simulink model "smib_53_start"  (Simulink 3.00)
settings: Solver=ode3  StartTime=0.0  StopTime=15  FixedStep=1e-4  MaxStep=1e-4  RelTol=1e-4
values from neighbouring files (symbols this model uses):
  D = 0.01    [MODEL_WORKSPACE.mat]    (also in MODEL_WORKSPACE_53.mat; WS.mat)
  J = 20    [MODEL_WORKSPACE.mat]    (also in MODEL_WORKSPACE_53.mat; WS.mat)
  Rf = 0.00246    [MODEL_WORKSPACE.mat]    (also in MODEL_WORKSPACE_53.mat = 0.0025; WS.mat = 0.0025)
  Tdo = 3    [MODEL_WORKSPACE.mat]    (also in MODEL_WORKSPACE_53.mat; WS.mat)
  X = 0.4    [MODEL_WORKSPACE.mat]    (also in MODEL_WORKSPACE_53.mat; WS.mat)
  Xd = 1    [MODEL_WORKSPACE.mat]    (also in MODEL_WORKSPACE_53.mat; WS.mat)
  Xdp = 0.25    [MODEL_WORKSPACE.mat]    (also in MODEL_WORKSPACE_53.mat; WS.mat)
  Xf = 0.8    [MODEL_WORKSPACE.mat]    (also in MODEL_WORKSPACE_53.mat; WS.mat)
libraries: simulink3 x1
settings Model: LastModifiedBy=FK

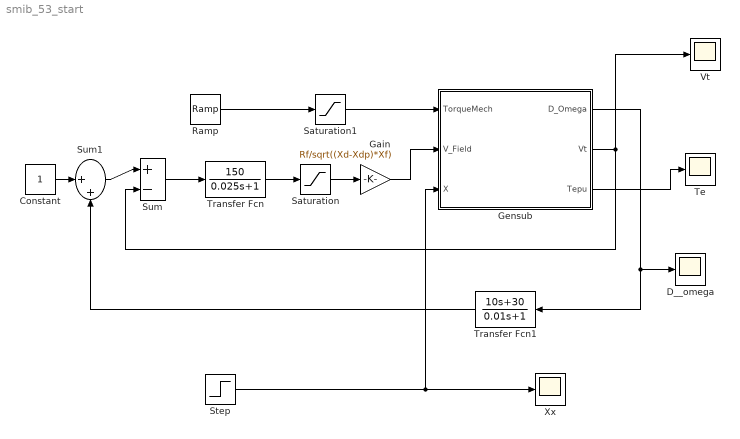
== system smib_53_start ==
  Constant : Constant  Value=1
  D__omega : Scope
      settings: TimeRange=auto  YMin=0  YMax=0.003  SaveToWorkspace=off  SaveName=ScopeData  MaxRows=500000
  Gain : Gain  Gain=Rf/sqrt((Xd-Xdp)*Xf)  SaturateOnIntegerOverflow=on
  Gensub : Subsystem
  Ramp : simulink3/Sources/Ramp  slope=0.3  start=0  X0=0
  Saturation : Saturate  UpperLimit=1.9  LowerLimit=0
  Saturation1 : Saturate  UpperLimit=1  LowerLimit=0
  Step : Step  Time=0.9  Before=10000*X  After=X  SampleTime=0
  Sum : Sum  Inputs=|+-  SaturateOnIntegerOverflow=on
  Sum1 : Sum  Inputs=|++  SaturateOnIntegerOverflow=on
  Te : Scope
      settings: TimeRange=auto  YMin=-0.5  YMax=1.5  SaveToWorkspace=off  SaveName=ScopeData  MaxRows=500000
  Transfer Fcn : TransferFcn  Numerator=[150]  Denominator=[0.025 1]
  Transfer Fcn1 : TransferFcn  Orientation=left  Numerator=[10 30]  Denominator=[0.01 1]
  Vt : Scope
      settings: TimeRange=auto  YMin=0  YMax=1.25  SaveToWorkspace=off  SaveName=ScopeData  MaxRows=500000
  Xx : Scope
      settings: TimeRange=auto  YMin=0  YMax=4000  SaveToWorkspace=off  SaveName=ScopeData  MaxRows=500000
  wires:
  Gain/1 -> Gensub/2(V_Field)
  Saturation/1 -> Gain/1
  Transfer Fcn/1 -> Saturation/1
  Sum/1 -> Transfer Fcn/1
  Sum1/1 -> Sum/1
  Constant/1 -> Sum1/1
  Gensub/2(Vt) -> Sum/2, Vt/1
  Gensub/3(Tepu) -> Te/1
  Ramp/1 -> Saturation1/1
  Saturation1/1 -> Gensub/1(TorqueMech)
  Gensub/1(D_Omega) -> D__omega/1, Transfer Fcn1/1
  Step/1 -> Gensub/3(X), Xx/1
  Transfer Fcn1/1 -> Sum1/2

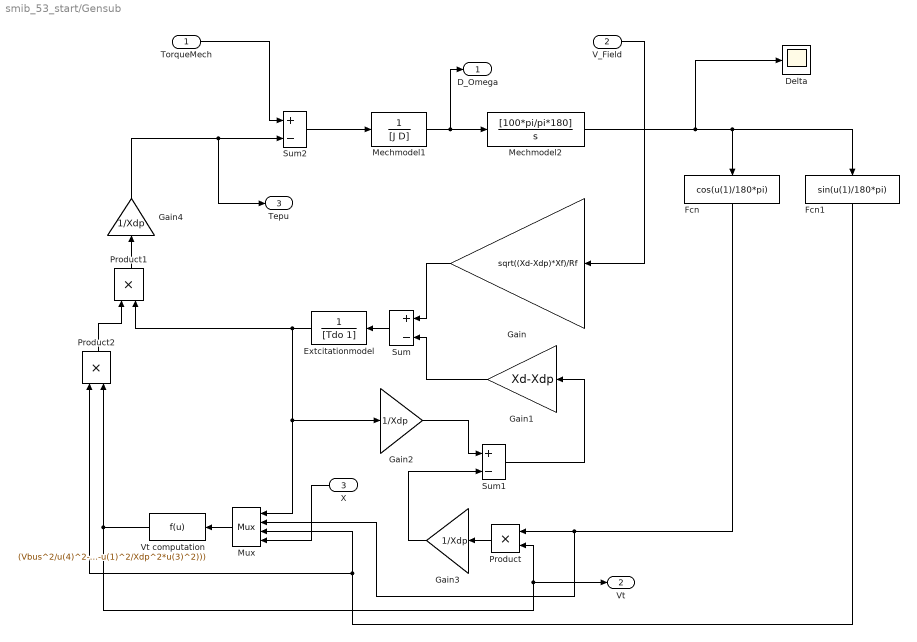
== system smib_53_start/Gensub ==
  TorqueMech : Inport  Port=1  PortWidth=-1  SampleTime=-1  DataType=auto
      settings: SignalType=auto
  V_Field : Inport  Port=2  PortWidth=-1  SampleTime=-1  DataType=auto
      settings: SignalType=auto
  X : Inport  Orientation=left  Port=3  PortWidth=-1  SampleTime=-1  DataType=auto
      settings: SignalType=auto
  Delta : Scope
      settings: TimeRange=auto  YMin=-10  YMax=60  SaveToWorkspace=off  SaveName=ScopeData  MaxRows=500000
  Extcitationmodel : TransferFcn  Orientation=left  Numerator=[1]  Denominator=[Tdo 1]
  Fcn : Fcn  Orientation=down  Expr=cos(u(1)/180*pi)
  Fcn1 : Fcn  Orientation=down  Expr=sin(u(1)/180*pi)
  Gain : Gain  Orientation=left  Gain=sqrt((Xd-Xdp)*Xf)/Rf  SaturateOnIntegerOverflow=on
  Gain1 : Gain  Orientation=left  Gain=Xd-Xdp  SaturateOnIntegerOverflow=on
  Gain2 : Gain  Gain=1/Xdp  SaturateOnIntegerOverflow=on
  Gain3 : Gain  Orientation=left  Gain=1/Xdp  SaturateOnIntegerOverflow=on
  Gain4 : Gain  Orientation=up  Gain=1/Xdp  SaturateOnIntegerOverflow=on
  Mechmodel1 : TransferFcn  Numerator=[1]  Denominator=[J D]
  Mechmodel2 : TransferFcn  Numerator=[100*pi/pi*180]  Denominator=[1 0]
  Mux : Mux  Orientation=left  Inputs=4
      settings: DisplayOption=none
  Product : Product  Orientation=left  Inputs=2  SaturateOnIntegerOverflow=on
  Product1 : Product  Orientation=up  Inputs=2  SaturateOnIntegerOverflow=on
  Product2 : Product  Orientation=up  Inputs=2  SaturateOnIntegerOverflow=on
  Sum : Sum  Orientation=left  Inputs=|+-  SaturateOnIntegerOverflow=on
  Sum1 : Sum  Inputs=|+-  SaturateOnIntegerOverflow=on
  Sum2 : Sum  Inputs=|+-  SaturateOnIntegerOverflow=on
  Vt computation : Fcn  Orientation=left  Expr=(Vbus^2/u(4)^2-u(1)^2/Xdp^2*u(3)^2>=0)*1/(1/u(4)+1/Xdp)*(u(1)/Xdp*u(2)+sqrt(abs(Vbus^2/u(4)^2-u(1)^2/Xdp^2*u(3)^2)))
  D_Omega : Outport  Port=1
  Vt : Outport  Port=2
  Tepu : Outport  Port=3
  wires:
  Mechmodel1/1 -> Mechmodel2/1, D_Omega/1
  V_Field/1 -> Gain/1
  Gain/1 -> Sum/1
  Gain1/1 -> Sum/2
  Sum1/1 -> Gain1/1
  Gain2/1 -> Sum1/1
  Gain3/1 -> Sum1/2
  Product/1 -> Gain3/1
  Sum/1 -> Extcitationmodel/1
  Extcitationmodel/1 -> Product1/2, Gain2/1, Mux/1
  Product2/1 -> Product1/1
  Fcn/1 -> Product/1, Mux/2
  Fcn1/1 -> Mux/3, Product2/1
  Vt computation/1 -> Product2/2, Product/2, Vt/1
  Product1/1 -> Gain4/1
  Sum2/1 -> Mechmodel1/1
  TorqueMech/1 -> Sum2/1
  Gain4/1 -> Sum2/2, Tepu/1
  X/1 -> Mux/4
  Mechmodel2/1 -> Fcn/1, Fcn1/1, Delta/1
  Mux/1 -> Vt computation/1
